simulink model "notLinModel_S"  (R2021b)
settings: Solver=ode45  StartTime=0.0  StopTime=1  MaxStep=0.5*10^-2  RelTol=1e-9
values from neighbouring files (symbols this model uses):
  A = [0 1; -k/mass-(4*C_magnetic*Ib^2)/(mass*gap^3) -c/mass]    [Operation_.m]
  B = [0 (4*C_magnetic*Ib)/(mass*gap^2)]'    [Operation_.m]
  c = 0.75    [Operation_.m]
  C = [1 0]    [Operation_.m]
  C_magnetic = 3.73e-6    (= 3.73e-06)    [Operation_.m]
  D = 0    [Operation_.m]
  gap = 3E-4    (= 0.0003)    [Operation_.m]
  k = 345.0    (= 345)    [Operation_.m]
  Kf = lqr(A',C',Vd,Vn)'    [Operation_.m]
  Kr = lqr(A,B,Q,R)    [Operation_.m]
  mass = k/(4.5*2*pi)^2    (= 0.431553189588)    [Operation_.m]
settings Model: Creator=danli  LastModifiedBy=danli
settings SolverCC: AlgebraicLoopSolver=TrustRegion
settings DataIOCC: ExternalInput=getinputstruct(op1)  InitialState=getstatestruct(op1)  LoadExternalInput=on  LoadInitialState=on
settings DebuggingCC: SFMachineParentedDataDiag=warning

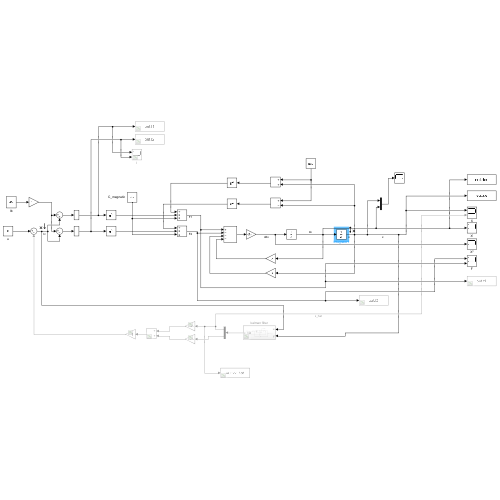
[thumbnail: Simulink's stored preview of the top-level diagram]
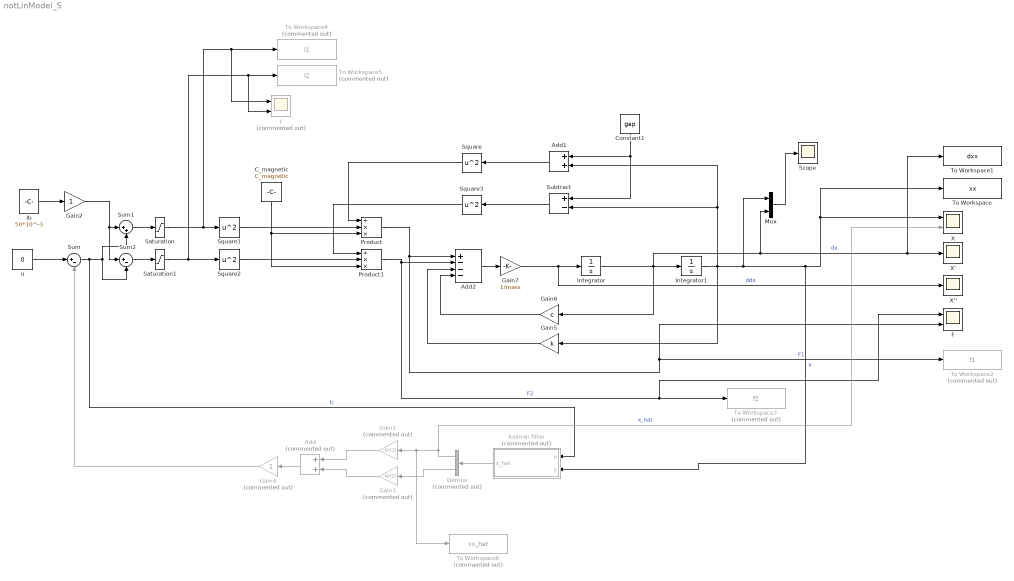
== system notLinModel_S ==
  Add : Sum  Commented=on
  Add1 : Sum
  Add2 : Sum  Inputs=+---
  C_magnetic : Constant  Value=C_magnetic
  Constant1 : Constant  Value=gap
  Demux : Demux  Commented=on  Outputs=2
  F : Scope  NumInputPorts=2
  Gain1 : Gain  Commented=on  Gain=Kr(1)
  Gain2 : Gain
  Gain3 : Gain  Commented=on  Gain=Kr(2)
  Gain4 : Gain  Commented=on
  Gain5 : Gain  Gain=k
  Gain6 : Gain  Gain=c
  Gain7 : Gain  Gain=1/mass
  I : Scope  Commented=on  NumInputPorts=2
  Ib : Constant  Value=50*10^-3
  Integrator : Integrator
  Integrator1 : Integrator
  Mux : Mux  Inputs=2
  Product : Product  Inputs=/**
  Product1 : Product  Inputs=/**
  Saturation : Saturate  UpperLimit=2  LowerLimit=0
  Saturation1 : Saturate  UpperLimit=2  LowerLimit=0
  Scope : Scope
  Square{,1..3} (4 alike) : Math  Operator=square  SaturateOnIntegerOverflow=on
  Subtract : Sum  Inputs=+-
  Sum : Sum  Inputs=|+-
  Sum1 : Sum  Inputs=|++
  Sum2 : Sum  Inputs=|+-
  To Workspace : ToWorkspace  VariableName=xx  SaveFormat=Timeseries  SampleTime=-1
  To Workspace1 : ToWorkspace  VariableName=dxx  SaveFormat=Timeseries  SampleTime=-1
  To Workspace2 : ToWorkspace  Commented=on  VariableName=f1  SaveFormat=Timeseries  SampleTime=-1
  To Workspace3 : ToWorkspace  Commented=on  VariableName=f2  SaveFormat=Timeseries  SampleTime=-1
  To Workspace4 : ToWorkspace  Commented=on  VariableName=I1  SaveFormat=Timeseries  SampleTime=-1
  To Workspace5 : ToWorkspace  Commented=on  VariableName=I2  SaveFormat=Timeseries  SampleTime=-1
  To Workspace6 : ToWorkspace  Commented=on  VariableName=xx_hat  SaveFormat=Timeseries  SampleTime=-1
  X : Scope  NumInputPorts=2
  X' : Scope
  X'' : Scope
  kalman filter : Subsystem  Commented=on
  u : Constant  Value=0
  wires:
  Ib/1 -> Gain2/1
  Sum1/1 -> Saturation/1
  Sum2/1 -> Saturation1/1
  Sum/1 -> kalman filter/1(u), Sum1/2, Sum2/2  "Ic"
  Gain2/1 -> Sum2/1, Sum1/1
  Add/1 -> Gain4/1
  Gain1/1 -> Add/1
  Gain3/1 -> Add/2
  Gain4/1 -> Sum/2
  Integrator1/1 -> Add1/2, Subtract/2, Mux/1, To Workspace/1, X/1, kalman filter/2(y), Gain5/1  "x"
  Saturation1/1 -> To Workspace5/1, I/2, Square2/1
  Saturation/1 -> I/1, To Workspace4/1, Square1/1
  Square2/1 -> Product1/2
  Constant1/1 -> Subtract/1, Add1/1
  Square1/1 -> Product/2
  Gain6/1 -> Add2/4
  Integrator/1 -> Gain6/1, Mux/2, To Workspace1/1, X'/1, Integrator1/1  "dx"
  Gain5/1 -> Add2/3
  Product1/1 -> F/1, To Workspace3/1, Add2/2  "F2"
  Subtract/1 -> Square3/1
  Square/1 -> Product/1
  Add1/1 -> Square/1
  Add2/1 -> Gain7/1
  Product/1 -> Add2/1, F/2, To Workspace2/1  "F1"
  Square3/1 -> Product1/1
  C_magnetic/1 -> Product/3, Product1/3
  Gain7/1 -> Integrator/1, X''/1  "ddx"
  kalman filter/1(x_hat) -> Demux/1
  Demux/2 -> Gain3/1
  Demux/1 -> X/2, To Workspace6/1, Gain1/1  "x_hat"
  u/1 -> Sum/1
  Mux/1 -> Scope/1

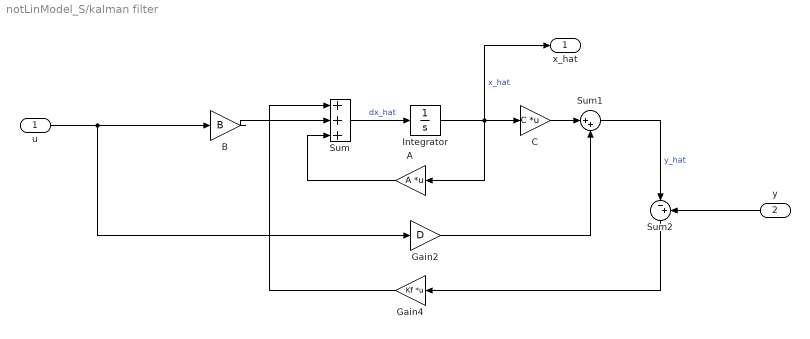
== system notLinModel_S/kalman filter ==
  u : Inport
  y : Inport  Port=2
  A : Gain  Gain=A  Multiplication=Matrix(K*u) (u vector)
  B : Gain  Gain=B
  C : Gain  Gain=C  Multiplication=Matrix(K*u) (u vector)
  Gain2 : Gain  Gain=D
  Gain4 : Gain  Gain=Kf  Multiplication=Matrix(K*u) (u vector)
  Integrator : Integrator  InitialCondition=[3*10^-5 0]
  Sum : Sum  Inputs=|+++
  Sum1 : Sum  Inputs=|++
  Sum2 : Sum  Inputs=|-+
  x_hat : Outport
  wires:
  Sum1/1 -> Sum2/1  "y_hat"
  Integrator/1 -> x_hat/1, A/1, C/1  "x_hat"
  Gain2/1 -> Sum1/2
  C/1 -> Sum1/1
  Sum/1 -> Integrator/1  "dx_hat"
  A/1 -> Sum/3
  y/1 -> Sum2/2
  Sum2/1 -> Gain4/1
  Gain4/1 -> Sum/1
  u/1 -> B/1, Gain2/1
  B/1 -> Sum/2
